simulink model "model3"  (R2022a)
settings: Solver=VariableStepAuto  StartTime=0.0  StopTime=8  RelTol=1e-3
undefined symbols (not defined in the file): A, B, C, K, L, x0, x_0
settings Model: Creator=Family  LastModifiedBy=Family

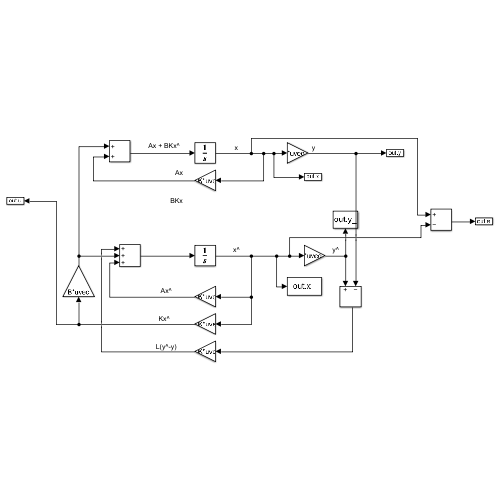
[thumbnail: Simulink's stored preview of the top-level diagram]
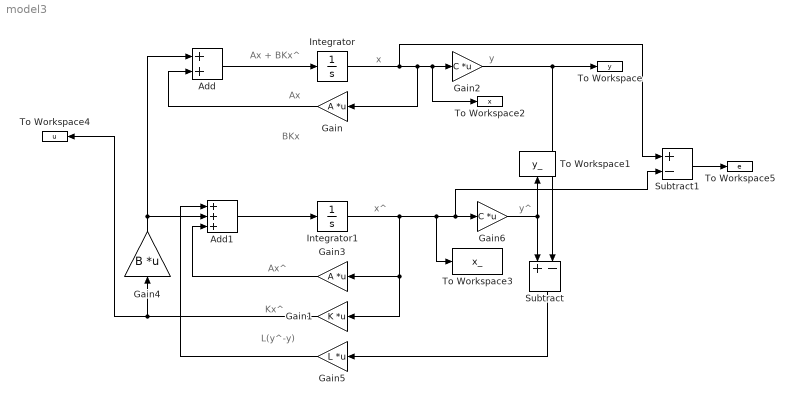
== system model3 ==
  note: L(y^-y)
  note: Kx^
  note: Ax + BKx^
  note: BKx
  note: x^
  note: Ax
  note: y^
  note: y
  note: x
  note: Ax^
  Add : Sum
  Add1 : Sum  Inputs=+++
  Gain : Gain  Gain=A  Multiplication=Matrix(K*u) (u vector)
  Gain1 : Gain  Gain=K  Multiplication=Matrix(K*u) (u vector)
  Gain2 : Gain  Gain=C  Multiplication=Matrix(K*u) (u vector)
  Gain3 : Gain  Gain=A  Multiplication=Matrix(K*u) (u vector)
  Gain4 : Gain  Gain=B  Multiplication=Matrix(K*u) (u vector)
  Gain5 : Gain  Gain=L  Multiplication=Matrix(K*u) (u vector)
  Gain6 : Gain  Gain=C  Multiplication=Matrix(K*u) (u vector)
  Integrator : Integrator  InitialCondition=x0
  Integrator1 : Integrator  InitialCondition=x_0
  Subtract : Sum  Inputs=+-
  Subtract1 : Sum  Inputs=+-
  To Workspace : ToWorkspace  VariableName=y  SaveFormat=Timeseries  SampleTime=0.0001
  To Workspace1 : ToWorkspace  VariableName=y_  SaveFormat=Timeseries  SampleTime=-1
  To Workspace2 : ToWorkspace  VariableName=x  SaveFormat=Timeseries  SampleTime=-1
  To Workspace3 : ToWorkspace  VariableName=x_  SaveFormat=Timeseries  SampleTime=-1
  To Workspace4 : ToWorkspace  VariableName=u  SaveFormat=Timeseries  SampleTime=-1
  To Workspace5 : ToWorkspace  VariableName=e  SaveFormat=Timeseries  SampleTime=-1
  wires:
  Gain4/1 -> Add1/2, Add/1
  Gain1/1 -> To Workspace4/1, Gain4/1
  Gain6/1 -> Subtract/1, To Workspace1/1
  Gain3/1 -> Add1/3
  Subtract1/1 -> To Workspace5/1
  Gain5/1 -> Add1/1
  Gain/1 -> Add/2
  Integrator1/1 -> Gain1/1, Gain3/1, To Workspace3/1, Subtract1/2, Gain6/1
  Gain2/1 -> To Workspace/1, Subtract/2
  Add1/1 -> Integrator1/1
  Subtract/1 -> Gain5/1
  Add/1 -> Integrator/1
  Integrator/1 -> Subtract1/1, To Workspace2/1, Gain2/1, Gain/1
